simulink model "window_size_alg_1"  (R2019b)
settings: Solver=ode45  StartTime=0.0  StopTime=0.03  MaxStep=1e-4  RelTol=1e-4  AbsTol=1e-6
settings Model: ExtModeTrigMode=oneshot  ExtModeArmWhenConnect=off  Creator=PC  LastModifiedBy=bae_rashid
settings SolverCC: AutoScaleAbsTol=off
settings DataIOCC: SaveFormat=Array  SignalLoggingSaveFormat=ModelDataLogs  ReturnWorkspaceOutputs=off
settings OptimizationCC: BlockReduction=off  BooleanDataType=off  LifeSpan=inf
settings DebuggingCC: SaveWithParameterizedLinksMsg=none  UnderspecifiedInitializationDetection=Classic  MergeDetectMultiDrivingBlocksExec=none  SignalResolutionControl=TryResolveAllWithWarning  MultiTaskDSMMsg=warning  MultiTaskCondExecSysMsg=none  SFUnexpectedBacktrackingDiag=warning  SFNoUnconditionalDefaultTransitionDiag=warning  SFExecutionAtInitializationDiag=none  ArithmeticOperatorsInVariantConditions=warning
settings HardwareCC: ProdBitPerPointer=32  ProdBitPerSizeT=32  ProdBitPerPtrDiffT=32  ProdLargestAtomicFloat=None  ProdIntDivRoundTo=Undefined  ProdEndianess=Unspecified  ProdWordSize=32  ProdHWDeviceType=32-bit Generic  TargetUnknown=on
settings ModelReferenceCC: PropagateSignalLabelsOutOfModel=off
settings SFSimCC: SimUseLocalCustomCode=off  CustomCodeUndefinedFunction=UseInterfaceOnly
settings RTWCC: TemplateMakefile=grt_vc.tmf  RTWUseLocalCustomCode=off
settings CodeAppCC: StateflowObjectComments=on
settings GRTTargetCC: TargetLangStandard=C89/C90 (ANSI)  GeneratePreprocessorConditionals=Disable all  CombineOutputUpdateFcns=off  GRTInterface=on
settings ConfigComp: CovMetricSettings=dw  CovHtmlReporting=on  CovSaveCumulativeToWorkspaceVar=on  CovSaveSingleToWorkspaceVar=on  CovExternalEMLEnable=off

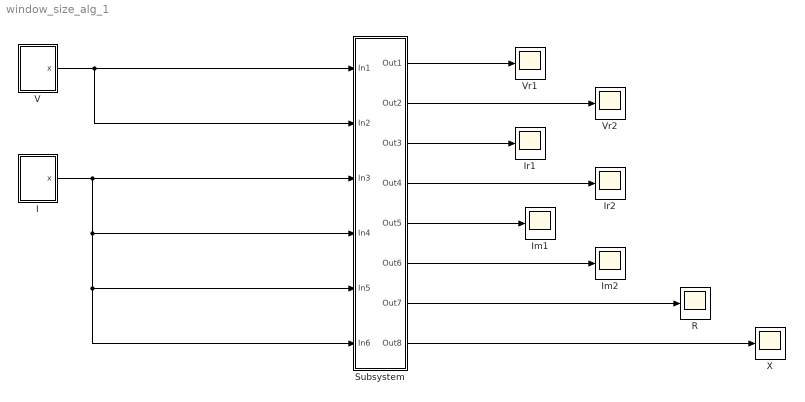
== system window_size_alg_1 ==
  I : Subsystem  mask(Signal Generator){A1=2, f1=60, A2=0, f2=2*60, A3=0, f3=5*60, tstart=1.5/60}
      mask prompts: A1 "Amplitude 1"; f1 "Frequency 1 [Hz]"; A2 "Amplitude 2"; f2 "Frequency 2 [Hz]"; A3 "Amplitude 3"; f3 "Frequency 3 [Hz]"; tstart "Start time [sec]"
  Im1 : Scope
  Im2 : Scope
  Ir1 : Scope
  Ir2 : Scope
  R : Scope
  Subsystem : Subsystem  mask{sr=60*60, ws_start=6, ws_end=6}
      mask prompts: sr "Sampling Rate [Hz]"; ws_start "Initial Window Size [# of Samples]"; ws_end "Final Window Size [# of Samples]"
  V : Subsystem  mask(Signal Generator){A1=10, f1=60, A2=0, f2=2*60, A3=0, f3=5*60, tstart=1.5/60, phase1=pi/4*1}
      mask prompts: A1 "Amplitude 1"; f1 "Frequency 1 [Hz]"; A2 "Amplitude 2"; f2 "Frequency 2 [Hz]"; A3 "Amplitude 3"; f3 "Frequency 3 [Hz]"; tstart "Start time [sec]"; phase1 "Phase 1"
  Vr1 : Scope
  Vr2 : Scope
  X : Scope
  wires:
  V/1(x) -> Subsystem/1(In1), Subsystem/2(In2)
  I/1(x) -> Subsystem/3(In3), Subsystem/6(In6), Subsystem/5(In5), Subsystem/4(In4)
  Subsystem/1(Out1) -> Vr1/1
  Subsystem/2(Out2) -> Vr2/1
  Subsystem/3(Out3) -> Ir1/1
  Subsystem/4(Out4) -> Ir2/1
  Subsystem/5(Out5) -> Im1/1
  Subsystem/6(Out6) -> Im2/1
  Subsystem/7(Out7) -> R/1
  Subsystem/8(Out8) -> X/1

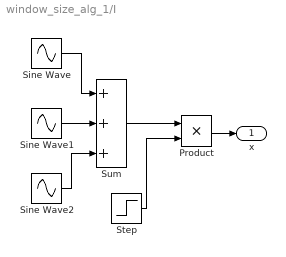
== system window_size_alg_1/I ==
  Product : Product  SaturateOnIntegerOverflow=on  RndMeth=Zero  InputSameDT=on  OutDataTypeStr=Inherit: Same as first input
  Sine Wave : Sin  Amplitude=A1  Frequency=f1*2*pi  SampleTime=0
  Sine Wave1 : Sin  Amplitude=A2  Frequency=f2*2*pi  SampleTime=0
  Sine Wave2 : Sin  Amplitude=A3  Frequency=f3*2*pi  SampleTime=0
  Step : Step  Time=tstart
  Sum : Sum  Inputs=+++  SaturateOnIntegerOverflow=on  InputSameDT=on  OutDataTypeStr=Inherit: Same as first input
  x : Outport  InitialOutput=0
  wires:
  Sine Wave/1 -> Sum/1
  Sine Wave1/1 -> Sum/2
  Sine Wave2/1 -> Sum/3
  Sum/1 -> Product/1
  Step/1 -> Product/2
  Product/1 -> x/1

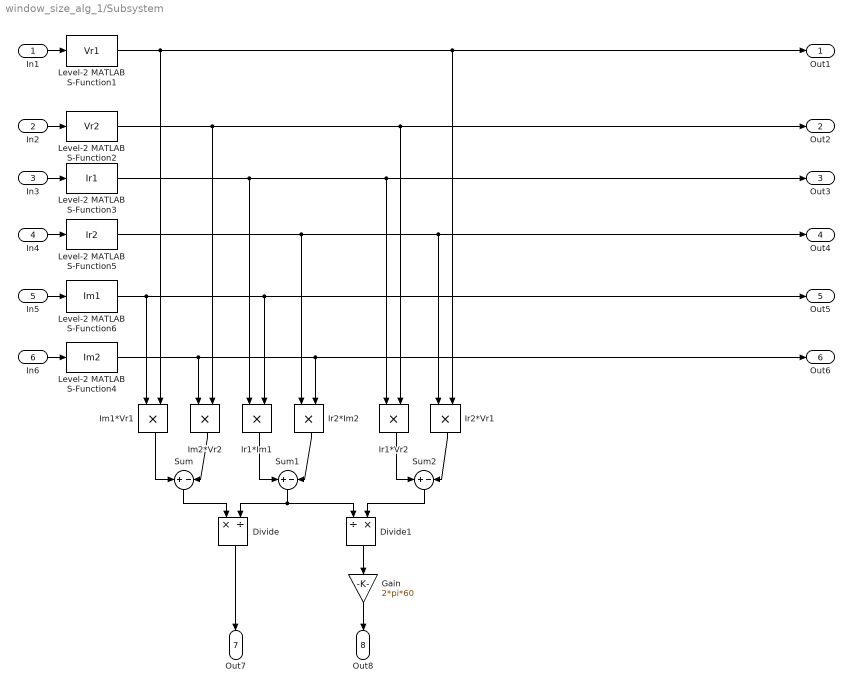
== system window_size_alg_1/Subsystem ==
  In1 : Inport
  In2 : Inport  Port=2
  In3 : Inport  Port=3
  In4 : Inport  Port=4
  In5 : Inport  Port=5
  In6 : Inport  Port=6
  Divide : Product  Inputs=*/
  Divide1 : Product  Inputs=/*
  Gain : Gain  Gain=2*pi*60
  Im1*Vr1 : Product  SaturateOnIntegerOverflow=on  RndMeth=Zero  InputSameDT=on  OutDataTypeStr=Inherit: Same as first input
  Im2*Vr2 : Product  SaturateOnIntegerOverflow=on  RndMeth=Zero  InputSameDT=on  OutDataTypeStr=Inherit: Same as first input
  Ir1*Im1 : Product  SaturateOnIntegerOverflow=on  RndMeth=Zero  InputSameDT=on  OutDataTypeStr=Inherit: Same as first input
  Ir1*Vr2 : Product  SaturateOnIntegerOverflow=on  RndMeth=Zero  InputSameDT=on  OutDataTypeStr=Inherit: Same as first input
  Ir2*Im2 : Product  SaturateOnIntegerOverflow=on  RndMeth=Zero  InputSameDT=on  OutDataTypeStr=Inherit: Same as first input
  Ir2*Vr1 : Product  SaturateOnIntegerOverflow=on  RndMeth=Zero  InputSameDT=on  OutDataTypeStr=Inherit: Same as first input
  Level-2 MATLAB S-Function1 : M-S-Function  FunctionName=Vr1  Parameters=sr,ws_start,ws_end
  Level-2 MATLAB S-Function2 : M-S-Function  FunctionName=Vr2  Parameters=sr,ws_start,ws_end
  Level-2 MATLAB S-Function3 : M-S-Function  FunctionName=Ir1  Parameters=sr,ws_start,ws_end
  Level-2 MATLAB S-Function4 : M-S-Function  FunctionName=Im2  Parameters=sr,ws_start,ws_end
  Level-2 MATLAB S-Function5 : M-S-Function  FunctionName=Ir2  Parameters=sr,ws_start,ws_end
  Level-2 MATLAB S-Function6 : M-S-Function  FunctionName=Im1  Parameters=sr,ws_start,ws_end
  Sum : Sum  Inputs=+-
  Sum1 : Sum  Inputs=+-
  Sum2 : Sum  Inputs=+-
  Out1 : Outport
  Out2 : Outport  Port=2
  Out3 : Outport  Port=3
  Out4 : Outport  Port=4
  Out5 : Outport  Port=5
  Out6 : Outport  Port=6
  Out7 : Outport  Port=7
  Out8 : Outport  Port=8
  wires:
  In2/1 -> Level-2 MATLAB S-Function2/1
  Level-2 MATLAB S-Function4/1 -> Im2*Vr2/1, Ir2*Im2/2, Out6/1
  In1/1 -> Level-2 MATLAB S-Function1/1
  In5/1 -> Level-2 MATLAB S-Function6/1
  Level-2 MATLAB S-Function6/1 -> Ir1*Im1/2, Out5/1, Im1*Vr1/1
  Level-2 MATLAB S-Function3/1 -> Ir1*Im1/1, Ir1*Vr2/1, Out3/1
  In3/1 -> Level-2 MATLAB S-Function3/1
  Level-2 MATLAB S-Function1/1 -> Ir2*Vr1/2, Out1/1, Im1*Vr1/2
  In4/1 -> Level-2 MATLAB S-Function5/1
  Level-2 MATLAB S-Function5/1 -> Ir2*Im2/1, Ir2*Vr1/1, Out4/1
  In6/1 -> Level-2 MATLAB S-Function4/1
  Level-2 MATLAB S-Function2/1 -> Im2*Vr2/2, Ir1*Vr2/2, Out2/1
  Im1*Vr1/1 -> Sum/1
  Im2*Vr2/1 -> Sum/2
  Ir1*Im1/1 -> Sum1/1
  Ir2*Im2/1 -> Sum1/2
  Sum/1 -> Divide/1
  Sum1/1 -> Divide/2, Divide1/1
  Divide/1 -> Out7/1
  Ir1*Vr2/1 -> Sum2/1
  Ir2*Vr1/1 -> Sum2/2
  Sum2/1 -> Divide1/2
  Divide1/1 -> Gain/1
  Gain/1 -> Out8/1

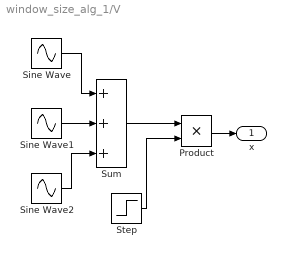
== system window_size_alg_1/V ==
  Product : Product  SaturateOnIntegerOverflow=on  RndMeth=Zero  InputSameDT=on  OutDataTypeStr=Inherit: Same as first input
  Sine Wave : Sin  Amplitude=A1  Frequency=f1*2*pi  Phase=phase1  SampleTime=0
  Sine Wave1 : Sin  Amplitude=A2  Frequency=f2*2*pi  SampleTime=0
  Sine Wave2 : Sin  Amplitude=A3  Frequency=f3*2*pi  SampleTime=0
  Step : Step  Time=tstart
  Sum : Sum  Inputs=+++  SaturateOnIntegerOverflow=on  InputSameDT=on  OutDataTypeStr=Inherit: Same as first input
  x : Outport  InitialOutput=0
  wires:
  Sine Wave/1 -> Sum/1
  Sine Wave1/1 -> Sum/2
  Sine Wave2/1 -> Sum/3
  Sum/1 -> Product/1
  Step/1 -> Product/2
  Product/1 -> x/1
